simulink model "abssq04_fixpt8_32"  (R2021b)
settings: Solver=VariableStepAuto  StartTime=0.0  StopTime=99  RelTol=1e-3
undefined symbols (not defined in the file or in its folder): figd2104, xcu250
libraries: hdlBasic x720, vmcUtilities x1
(part 5 of 7)

== system abssq04_fixpt8_32/total32/Subsystem25bit ==
  rex : Inport
  imx : Inport  Port=2
  CMult1 : hdlBasic/CMult  const=cos(pi/4)  gui_display_data_type=Fixed-point  const_n_bits=25  const_bin_pt=24  float_type=Single  exp_bits=8  fraction_bits=24  en=off  latency=0  precision=Full  arith_type="Signed  (2's comp)"  n_bits=16  bin_pt=14  quantization=Truncate  overflow=Wrap  use_behavioral_HDL=off  mem_type=Distributed RAM  pipeline=off  XmcBlockStatus=1  maskContainerNames=tabcontainer1  block_type=cmult  block_config=sysgen:CMult_config
      settings: infoedit=[]
  CMult2 : hdlBasic/CMult  const=cos(pi/4)  gui_display_data_type=Fixed-point  const_n_bits=25  const_bin_pt=24  float_type=Single  exp_bits=8  fraction_bits=24  en=off  latency=0  precision=Full  arith_type="Signed  (2's comp)"  n_bits=16  bin_pt=14  quantization=Truncate  overflow=Wrap  use_behavioral_HDL=off  mem_type=Distributed RAM  pipeline=off  XmcBlockStatus=1  maskContainerNames=tabcontainer1  block_type=cmult  block_config=sysgen:CMult_config
      settings: infoedit=[]
  CMult3 : hdlBasic/CMult  const=1/sqrt(2)  gui_display_data_type=Fixed-point  const_n_bits=25  const_bin_pt=24  float_type=Single  exp_bits=8  fraction_bits=24  en=off  latency=0  precision=Full  arith_type="Signed  (2's comp)"  n_bits=16  bin_pt=14  quantization=Truncate  overflow=Wrap  use_behavioral_HDL=off  mem_type=Distributed RAM  pipeline=off  XmcBlockStatus=1  maskContainerNames=tabcontainer1  block_type=cmult  block_config=sysgen:CMult_config
      settings: infoedit=[]
  COS_PI : hdlBasic/Constant  Commented=on  const=cos(pi/4)  gui_display_data_type=Fixed-point  arith_type=Unsigned  n_bits=8  bin_pt=7  preci_type=Double  exp_width=8  frac_width=24  explicit_period=on  period=1  XmcBlockStatus=1  maskContainerNames=tabcontainer1  block_type=constant  block_config=sysgen:Constant_config
  Cast1 : hdlBasic/Convert  Commented=on  gui_display_data_type=Fixed-point  arith_type=Unsigned  n_bits=8  bin_pt=7  float_type=Double  exp_bits=8  fraction_bits=24  quantization="Round  (unbiased: +/- Inf)"  overflow=Saturate  en=off  latency=0  pipeline=on  XmcBlockStatus=1  maskContainerNames=group2  block_type=convert  block_config=sysgen:Convert_config
  Cast2 : hdlBasic/Convert  Commented=on  gui_display_data_type=Fixed-point  arith_type=Unsigned  n_bits=8  bin_pt=7  float_type=Double  exp_bits=8  fraction_bits=24  quantization="Round  (unbiased: +/- Inf)"  overflow=Saturate  en=off  latency=0  pipeline=on  XmcBlockStatus=1  maskContainerNames=group2  block_type=convert  block_config=sysgen:Convert_config
  Cast3 : hdlBasic/Convert  Commented=on  gui_display_data_type=Fixed-point  arith_type=Unsigned  n_bits=8  bin_pt=7  float_type=Double  exp_bits=8  fraction_bits=24  quantization="Round  (unbiased: +/- Inf)"  overflow=Saturate  en=off  latency=0  pipeline=on  XmcBlockStatus=1  maskContainerNames=group2  block_type=convert  block_config=sysgen:Convert_config
  Gate_In1 : hdlBasic/Gateway In  gui_display_data_type=Fixed-point  arith_type=Signed (2's comp)  n_bits=25  bin_pt=23  preci_type=Double  exp_width=8  frac_width=24  rows=1  columns=1  quantization=Truncate  overflow=Wrap  period=1  UseAsADC=off  ADCChannel='1'  interface=None  automatic_assignment=on  address_offset=hex2dec('00')  intf_name=''  intf_description=''  default_value=0  timing_constraint=None  locs_specified=off  LOCs={}  io_standard={}  inherit_from_input=off  hdl_port=on  XmcBlockStatus=1  maskContainerNames=group4  block_type=gatewayin  block_config=sysgen:gateway_in_config  block_width_w=590  block_height_w=620  block_width=640  block_height=850
  Gate_In2 : hdlBasic/Gateway In  gui_display_data_type=Fixed-point  arith_type=Signed (2's comp)  n_bits=25  bin_pt=23  preci_type=Double  exp_width=8  frac_width=24  rows=1  columns=1  quantization=Truncate  overflow=Wrap  period=1  UseAsADC=off  ADCChannel='1'  interface=None  automatic_assignment=on  address_offset=hex2dec('00')  intf_name=''  intf_description=''  default_value=0  timing_constraint=None  locs_specified=off  LOCs={}  io_standard={}  inherit_from_input=off  hdl_port=on  XmcBlockStatus=1  maskContainerNames=group4  block_type=gatewayin  block_config=sysgen:gateway_in_config  block_width_w=590  block_height_w=620  block_width=640  block_height=850
  Gate_out1 : hdlBasic/Gateway Out  inherit_from_input=off  hdl_port=on  rows=1  columns=1  UseAsDAC=off  DACChannel='1'  interface=None  automatic_assignment=on  address_offset=hex2dec('00')  intf_name=''  intf_description=''  timing_constraint=None  locs_specified=off  LOCs={}  io_standard={}  XmcBlockStatus=1  maskContainerNames=group4  block_type=gatewayout  block_config=sysgen:gateway_out_config  block_width_w=590  block_height_w=620  block_width=620  block_height=750
  Mux : hdlBasic/Mux  inputs=2  en=off  latency=0  precision=Full  arith_type=Unsigned  n_bits=16  bin_pt=14  quantization=Truncate  overflow=Wrap  XmcBlockStatus=1  maskContainerNames=tabcontainer1  block_type=mux  block_config=sysgen:Mux_config
  Scale1 : hdlBasic/Scale  scale_factor=-24  XmcBlockStatus=1  maskContainerNames=group1  block_type=scale  block_config=sysgen:Scale_config
  Scale2 : hdlBasic/Scale  scale_factor=-23  XmcBlockStatus=1  maskContainerNames=group1  block_type=scale  block_config=sysgen:Scale_config
  Scale3 : hdlBasic/Scale  scale_factor=-24  XmcBlockStatus=1  maskContainerNames=group1  block_type=scale  block_config=sysgen:Scale_config
  Slice1 : hdlBasic/Slice  nbits=8  boolean_output=off  mode=Two Bit Locations  bit1=-1  base1=MSB of Input  bit0=24  base0=LSB of Input  XmcBlockStatus=1  maskContainerNames=group1  block_type=slice  block_config=sysgen:Slice_config
  Slice2 : hdlBasic/Slice  nbits=24  boolean_output=off  mode=Upper Bit Location + Width  bit1=-3  base1=MSB of Input  bit0=7  base0=LSB of Input  XmcBlockStatus=1  maskContainerNames=group1  block_type=slice  block_config=sysgen:Slice_config
  Slice3 : hdlBasic/Slice  nbits=7  boolean_output=off  mode=Two Bit Locations  bit1=-5  base1=MSB of Input  bit0=23  base0=LSB of Input  XmcBlockStatus=1  maskContainerNames=group1  block_type=slice  block_config=sysgen:Slice_config
  abs{1..4} (4 alike) : hdlBasic/Absolute  precision=Full  arith_type=Unsigned  n_bits=16  bin_pt=14  quantization=Truncate  overflow=Wrap  en=off  latency=0  XmcBlockStatus=1  maskContainerNames=tabcontainer1  block_type=abs  block_config=sysgen:Abs_config
  addsub1 : hdlBasic/AddSub  mode=Subtraction  use_carryin=off  use_carryout=off  en=off  latency=0  precision=Full  arith_type="Signed  (2's comp)"  n_bits=35  bin_pt=32  quantization="Round  (unbiased: +/- Inf)"  overflow=Saturate  use_behavioral_HDL=off  hw_selection=Fabric  pipelined=on  XmcBlockStatus=1  maskContainerNames=tabcontainer1  block_type=addsub  block_config=sysgen:Addsub_config
  addsub2 : hdlBasic/AddSub  mode=Addition  use_carryin=off  use_carryout=off  en=off  latency=0  precision=Full  arith_type=Unsigned  n_bits=16  bin_pt=14  quantization="Round  (unbiased: +/- Inf)"  overflow=Saturate  use_behavioral_HDL=off  hw_selection=Fabric  pipelined=on  XmcBlockStatus=1  maskContainerNames=tabcontainer1  block_type=addsub  block_config=sysgen:Addsub_config
  addsub3 : hdlBasic/AddSub  mode=Addition  use_carryin=off  use_carryout=off  en=off  latency=0  precision=Full  arith_type=Unsigned  n_bits=16  bin_pt=14  quantization="Round  (unbiased: +/- Inf)"  overflow=Saturate  use_behavioral_HDL=off  hw_selection=Fabric  pipelined=on  XmcBlockStatus=1  maskContainerNames=tabcontainer1  block_type=addsub  block_config=sysgen:Addsub_config
  addsub4 : hdlBasic/AddSub  mode=Addition  use_carryin=off  use_carryout=off  en=off  latency=0  precision=Full  arith_type=Unsigned  n_bits=17  bin_pt=16  quantization="Round  (unbiased: +/- Inf)"  overflow=Saturate  use_behavioral_HDL=off  hw_selection=Fabric  pipelined=on  XmcBlockStatus=1  maskContainerNames=tabcontainer1  block_type=addsub  block_config=sysgen:Addsub_config
  bool1 : hdlBasic/Relational  mode=a<b  op_type=Bool  en=off  latency=0  XmcBlockStatus=1  maskContainerNames=tabcontainer1  block_type=relational  block_config=sysgen:Relational_config
  mult1 : hdlBasic/Mult  Commented=on  precision=Full  arith_type=Unsigned  n_bits=32  bin_pt=32  quantization="Round  (unbiased: +/- Inf)"  overflow=Saturate  en=off  latency=0  use_behavioral_HDL=off  opt=Area  use_embedded=off  optimum_pipeline=off  pipeline=on  use_rpm=on  placement_style=Triangular  XmcBlockStatus=1  maskContainerNames=group1  block_type=mult  block_config=sysgen:Mult_config
  mult2 : hdlBasic/Mult  Commented=on  precision=Full  arith_type=Unsigned  n_bits=32  bin_pt=32  quantization="Round  (unbiased: +/- Inf)"  overflow=Saturate  en=off  latency=0  use_behavioral_HDL=off  opt=Area  use_embedded=off  optimum_pipeline=off  pipeline=on  use_rpm=on  placement_style=Triangular  XmcBlockStatus=1  maskContainerNames=group1  block_type=mult  block_config=sysgen:Mult_config
  mult3 : hdlBasic/Mult  Commented=on  precision=Full  arith_type="Signed  (2's comp)"  n_bits=16  bin_pt=14  quantization="Round  (unbiased: +/- Inf)"  overflow=Saturate  en=off  latency=0  use_behavioral_HDL=off  opt=Area  use_embedded=off  optimum_pipeline=off  pipeline=on  use_rpm=on  placement_style=Triangular  XmcBlockStatus=1  maskContainerNames=group1  block_type=mult  block_config=sysgen:Mult_config
  Out1 : Outport
  wires:
  addsub1/1 -> abs1/1
  abs1/1 -> addsub3/1
  CMult1/1 -> addsub2/1, addsub1/1
  CMult2/1 -> addsub2/2, addsub1/2
  CMult3/1 -> Slice1/1
  Mux/1 -> CMult3/1
  imx/1 -> Gate_In2/1
  Gate_out1/1 -> Out1/1
  rex/1 -> Gate_In1/1
  Slice1/1 -> Scale1/1
  bool1/1 -> Mux/1
  addsub3/1 -> Slice3/1
  addsub4/1 -> Slice2/1
  addsub2/1 -> abs2/1
  Gate_In2/1 -> abs4/1, CMult2/1
  Gate_In1/1 -> CMult1/1, abs3/1
  abs2/1 -> addsub3/2
  abs3/1 -> addsub4/1
  abs4/1 -> addsub4/2
  Scale1/1 -> Gate_out1/1
  Slice2/1 -> Scale2/1
  Scale3/1 -> bool1/1, Mux/2
  Scale2/1 -> Mux/3, bool1/2
  Slice3/1 -> Scale3/1

== system abssq04_fixpt8_32/total32/Subsystem26bit ==
  rex : Inport
  imx : Inport  Port=2
  CMult1 : hdlBasic/CMult  const=cos(pi/4)  gui_display_data_type=Fixed-point  const_n_bits=26  const_bin_pt=25  float_type=Single  exp_bits=8  fraction_bits=24  en=off  latency=0  precision=Full  arith_type="Signed  (2's comp)"  n_bits=16  bin_pt=14  quantization=Truncate  overflow=Wrap  use_behavioral_HDL=off  mem_type=Distributed RAM  pipeline=off  XmcBlockStatus=1  maskContainerNames=tabcontainer1  block_type=cmult  block_config=sysgen:CMult_config
      settings: infoedit=[]
  CMult2 : hdlBasic/CMult  const=cos(pi/4)  gui_display_data_type=Fixed-point  const_n_bits=26  const_bin_pt=25  float_type=Single  exp_bits=8  fraction_bits=24  en=off  latency=0  precision=Full  arith_type="Signed  (2's comp)"  n_bits=16  bin_pt=14  quantization=Truncate  overflow=Wrap  use_behavioral_HDL=off  mem_type=Distributed RAM  pipeline=off  XmcBlockStatus=1  maskContainerNames=tabcontainer1  block_type=cmult  block_config=sysgen:CMult_config
      settings: infoedit=[]
  CMult3 : hdlBasic/CMult  const=1/sqrt(2)  gui_display_data_type=Fixed-point  const_n_bits=26  const_bin_pt=25  float_type=Single  exp_bits=8  fraction_bits=24  en=off  latency=0  precision=Full  arith_type="Signed  (2's comp)"  n_bits=16  bin_pt=14  quantization=Truncate  overflow=Wrap  use_behavioral_HDL=off  mem_type=Distributed RAM  pipeline=off  XmcBlockStatus=1  maskContainerNames=tabcontainer1  block_type=cmult  block_config=sysgen:CMult_config
      settings: infoedit=[]
  COS_PI : hdlBasic/Constant  Commented=on  const=cos(pi/4)  gui_display_data_type=Fixed-point  arith_type=Unsigned  n_bits=8  bin_pt=7  preci_type=Double  exp_width=8  frac_width=24  explicit_period=on  period=1  XmcBlockStatus=1  maskContainerNames=tabcontainer1  block_type=constant  block_config=sysgen:Constant_config
  Cast1 : hdlBasic/Convert  Commented=on  gui_display_data_type=Fixed-point  arith_type=Unsigned  n_bits=8  bin_pt=7  float_type=Double  exp_bits=8  fraction_bits=24  quantization="Round  (unbiased: +/- Inf)"  overflow=Saturate  en=off  latency=0  pipeline=on  XmcBlockStatus=1  maskContainerNames=group2  block_type=convert  block_config=sysgen:Convert_config
  Cast2 : hdlBasic/Convert  Commented=on  gui_display_data_type=Fixed-point  arith_type=Unsigned  n_bits=8  bin_pt=7  float_type=Double  exp_bits=8  fraction_bits=24  quantization="Round  (unbiased: +/- Inf)"  overflow=Saturate  en=off  latency=0  pipeline=on  XmcBlockStatus=1  maskContainerNames=group2  block_type=convert  block_config=sysgen:Convert_config
  Cast3 : hdlBasic/Convert  Commented=on  gui_display_data_type=Fixed-point  arith_type=Unsigned  n_bits=8  bin_pt=7  float_type=Double  exp_bits=8  fraction_bits=24  quantization="Round  (unbiased: +/- Inf)"  overflow=Saturate  en=off  latency=0  pipeline=on  XmcBlockStatus=1  maskContainerNames=group2  block_type=convert  block_config=sysgen:Convert_config
  Gate_In1 : hdlBasic/Gateway In  gui_display_data_type=Fixed-point  arith_type=Signed (2's comp)  n_bits=26  bin_pt=24  preci_type=Double  exp_width=8  frac_width=24  rows=1  columns=1  quantization=Truncate  overflow=Wrap  period=1  UseAsADC=off  ADCChannel='1'  interface=None  automatic_assignment=on  address_offset=hex2dec('00')  intf_name=''  intf_description=''  default_value=0  timing_constraint=None  locs_specified=off  LOCs={}  io_standard={}  inherit_from_input=off  hdl_port=on  XmcBlockStatus=1  maskContainerNames=group4  block_type=gatewayin  block_config=sysgen:gateway_in_config  block_width_w=590  block_height_w=620  block_width=640  block_height=850
  Gate_In2 : hdlBasic/Gateway In  gui_display_data_type=Fixed-point  arith_type=Signed (2's comp)  n_bits=26  bin_pt=24  preci_type=Double  exp_width=8  frac_width=24  rows=1  columns=1  quantization=Truncate  overflow=Wrap  period=1  UseAsADC=off  ADCChannel='1'  interface=None  automatic_assignment=on  address_offset=hex2dec('00')  intf_name=''  intf_description=''  default_value=0  timing_constraint=None  locs_specified=off  LOCs={}  io_standard={}  inherit_from_input=off  hdl_port=on  XmcBlockStatus=1  maskContainerNames=group4  block_type=gatewayin  block_config=sysgen:gateway_in_config  block_width_w=590  block_height_w=620  block_width=640  block_height=850
  Gate_out1 : hdlBasic/Gateway Out  inherit_from_input=off  hdl_port=on  rows=1  columns=1  UseAsDAC=off  DACChannel='1'  interface=None  automatic_assignment=on  address_offset=hex2dec('00')  intf_name=''  intf_description=''  timing_constraint=None  locs_specified=off  LOCs={}  io_standard={}  XmcBlockStatus=1  maskContainerNames=group4  block_type=gatewayout  block_config=sysgen:gateway_out_config  block_width_w=590  block_height_w=620  block_width=620  block_height=750
  Mux : hdlBasic/Mux  inputs=2  en=off  latency=0  precision=Full  arith_type=Unsigned  n_bits=16  bin_pt=14  quantization=Truncate  overflow=Wrap  XmcBlockStatus=1  maskContainerNames=tabcontainer1  block_type=mux  block_config=sysgen:Mux_config
  Scale1 : hdlBasic/Scale  scale_factor=-25  XmcBlockStatus=1  maskContainerNames=group1  block_type=scale  block_config=sysgen:Scale_config
  Scale2 : hdlBasic/Scale  scale_factor=-24  XmcBlockStatus=1  maskContainerNames=group1  block_type=scale  block_config=sysgen:Scale_config
  Scale3 : hdlBasic/Scale  scale_factor=-25  XmcBlockStatus=1  maskContainerNames=group1  block_type=scale  block_config=sysgen:Scale_config
  Slice1 : hdlBasic/Slice  nbits=8  boolean_output=off  mode=Two Bit Locations  bit1=-1  base1=MSB of Input  bit0=25  base0=LSB of Input  XmcBlockStatus=1  maskContainerNames=group1  block_type=slice  block_config=sysgen:Slice_config
  Slice2 : hdlBasic/Slice  nbits=25  boolean_output=off  mode=Upper Bit Location + Width  bit1=-3  base1=MSB of Input  bit0=7  base0=LSB of Input  XmcBlockStatus=1  maskContainerNames=group1  block_type=slice  block_config=sysgen:Slice_config
  Slice3 : hdlBasic/Slice  nbits=7  boolean_output=off  mode=Two Bit Locations  bit1=-5  base1=MSB of Input  bit0=24  base0=LSB of Input  XmcBlockStatus=1  maskContainerNames=group1  block_type=slice  block_config=sysgen:Slice_config
  abs{1..4} (4 alike) : hdlBasic/Absolute  precision=Full  arith_type=Unsigned  n_bits=16  bin_pt=14  quantization=Truncate  overflow=Wrap  en=off  latency=0  XmcBlockStatus=1  maskContainerNames=tabcontainer1  block_type=abs  block_config=sysgen:Abs_config
  addsub1 : hdlBasic/AddSub  mode=Subtraction  use_carryin=off  use_carryout=off  en=off  latency=0  precision=Full  arith_type="Signed  (2's comp)"  n_bits=35  bin_pt=32  quantization="Round  (unbiased: +/- Inf)"  overflow=Saturate  use_behavioral_HDL=off  hw_selection=Fabric  pipelined=on  XmcBlockStatus=1  maskContainerNames=tabcontainer1  block_type=addsub  block_config=sysgen:Addsub_config
  addsub2 : hdlBasic/AddSub  mode=Addition  use_carryin=off  use_carryout=off  en=off  latency=0  precision=Full  arith_type=Unsigned  n_bits=16  bin_pt=14  quantization="Round  (unbiased: +/- Inf)"  overflow=Saturate  use_behavioral_HDL=off  hw_selection=Fabric  pipelined=on  XmcBlockStatus=1  maskContainerNames=tabcontainer1  block_type=addsub  block_config=sysgen:Addsub_config
  addsub3 : hdlBasic/AddSub  mode=Addition  use_carryin=off  use_carryout=off  en=off  latency=0  precision=Full  arith_type=Unsigned  n_bits=16  bin_pt=14  quantization="Round  (unbiased: +/- Inf)"  overflow=Saturate  use_behavioral_HDL=off  hw_selection=Fabric  pipelined=on  XmcBlockStatus=1  maskContainerNames=tabcontainer1  block_type=addsub  block_config=sysgen:Addsub_config
  addsub4 : hdlBasic/AddSub  mode=Addition  use_carryin=off  use_carryout=off  en=off  latency=0  precision=Full  arith_type=Unsigned  n_bits=17  bin_pt=16  quantization="Round  (unbiased: +/- Inf)"  overflow=Saturate  use_behavioral_HDL=off  hw_selection=Fabric  pipelined=on  XmcBlockStatus=1  maskContainerNames=tabcontainer1  block_type=addsub  block_config=sysgen:Addsub_config
  bool1 : hdlBasic/Relational  mode=a<b  op_type=Bool  en=off  latency=0  XmcBlockStatus=1  maskContainerNames=tabcontainer1  block_type=relational  block_config=sysgen:Relational_config
  mult1 : hdlBasic/Mult  Commented=on  precision=Full  arith_type=Unsigned  n_bits=32  bin_pt=32  quantization="Round  (unbiased: +/- Inf)"  overflow=Saturate  en=off  latency=0  use_behavioral_HDL=off  opt=Area  use_embedded=off  optimum_pipeline=off  pipeline=on  use_rpm=on  placement_style=Triangular  XmcBlockStatus=1  maskContainerNames=group1  block_type=mult  block_config=sysgen:Mult_config
  mult2 : hdlBasic/Mult  Commented=on  precision=Full  arith_type=Unsigned  n_bits=32  bin_pt=32  quantization="Round  (unbiased: +/- Inf)"  overflow=Saturate  en=off  latency=0  use_behavioral_HDL=off  opt=Area  use_embedded=off  optimum_pipeline=off  pipeline=on  use_rpm=on  placement_style=Triangular  XmcBlockStatus=1  maskContainerNames=group1  block_type=mult  block_config=sysgen:Mult_config
  mult3 : hdlBasic/Mult  Commented=on  precision=Full  arith_type="Signed  (2's comp)"  n_bits=16  bin_pt=14  quantization="Round  (unbiased: +/- Inf)"  overflow=Saturate  en=off  latency=0  use_behavioral_HDL=off  opt=Area  use_embedded=off  optimum_pipeline=off  pipeline=on  use_rpm=on  placement_style=Triangular  XmcBlockStatus=1  maskContainerNames=group1  block_type=mult  block_config=sysgen:Mult_config
  Out1 : Outport
  wires:
  addsub1/1 -> abs1/1
  abs1/1 -> addsub3/1
  CMult1/1 -> addsub2/1, addsub1/1
  CMult2/1 -> addsub2/2, addsub1/2
  CMult3/1 -> Slice1/1
  Mux/1 -> CMult3/1
  imx/1 -> Gate_In2/1
  Gate_out1/1 -> Out1/1
  rex/1 -> Gate_In1/1
  Slice1/1 -> Scale1/1
  bool1/1 -> Mux/1
  addsub3/1 -> Slice3/1
  addsub4/1 -> Slice2/1
  addsub2/1 -> abs2/1
  Gate_In2/1 -> abs4/1, CMult2/1
  Gate_In1/1 -> CMult1/1, abs3/1
  abs2/1 -> addsub3/2
  abs3/1 -> addsub4/1
  abs4/1 -> addsub4/2
  Scale1/1 -> Gate_out1/1
  Slice2/1 -> Scale2/1
  Scale3/1 -> bool1/1, Mux/2
  Scale2/1 -> Mux/3, bool1/2
  Slice3/1 -> Scale3/1

== system abssq04_fixpt8_32/total32/Subsystem27bit ==
  rex : Inport
  imx : Inport  Port=2
  CMult1 : hdlBasic/CMult  const=cos(pi/4)  gui_display_data_type=Fixed-point  const_n_bits=27  const_bin_pt=26  float_type=Single  exp_bits=8  fraction_bits=24  en=off  latency=0  precision=Full  arith_type="Signed  (2's comp)"  n_bits=16  bin_pt=14  quantization=Truncate  overflow=Wrap  use_behavioral_HDL=off  mem_type=Distributed RAM  pipeline=off  XmcBlockStatus=1  maskContainerNames=tabcontainer1  block_type=cmult  block_config=sysgen:CMult_config
      settings: infoedit=[]
  CMult2 : hdlBasic/CMult  const=cos(pi/4)  gui_display_data_type=Fixed-point  const_n_bits=27  const_bin_pt=26  float_type=Single  exp_bits=8  fraction_bits=24  en=off  latency=0  precision=Full  arith_type="Signed  (2's comp)"  n_bits=16  bin_pt=14  quantization=Truncate  overflow=Wrap  use_behavioral_HDL=off  mem_type=Distributed RAM  pipeline=off  XmcBlockStatus=1  maskContainerNames=tabcontainer1  block_type=cmult  block_config=sysgen:CMult_config
      settings: infoedit=[]
  CMult3 : hdlBasic/CMult  const=1/sqrt(2)  gui_display_data_type=Fixed-point  const_n_bits=27  const_bin_pt=26  float_type=Single  exp_bits=8  fraction_bits=24  en=off  latency=0  precision=Full  arith_type="Signed  (2's comp)"  n_bits=16  bin_pt=14  quantization=Truncate  overflow=Wrap  use_behavioral_HDL=off  mem_type=Distributed RAM  pipeline=off  XmcBlockStatus=1  maskContainerNames=tabcontainer1  block_type=cmult  block_config=sysgen:CMult_config
      settings: infoedit=[]
  COS_PI : hdlBasic/Constant  Commented=on  const=cos(pi/4)  gui_display_data_type=Fixed-point  arith_type=Unsigned  n_bits=8  bin_pt=7  preci_type=Double  exp_width=8  frac_width=24  explicit_period=on  period=1  XmcBlockStatus=1  maskContainerNames=tabcontainer1  block_type=constant  block_config=sysgen:Constant_config
  Cast1 : hdlBasic/Convert  Commented=on  gui_display_data_type=Fixed-point  arith_type=Unsigned  n_bits=8  bin_pt=7  float_type=Double  exp_bits=8  fraction_bits=24  quantization="Round  (unbiased: +/- Inf)"  overflow=Saturate  en=off  latency=0  pipeline=on  XmcBlockStatus=1  maskContainerNames=group2  block_type=convert  block_config=sysgen:Convert_config
  Cast2 : hdlBasic/Convert  Commented=on  gui_display_data_type=Fixed-point  arith_type=Unsigned  n_bits=8  bin_pt=7  float_type=Double  exp_bits=8  fraction_bits=24  quantization="Round  (unbiased: +/- Inf)"  overflow=Saturate  en=off  latency=0  pipeline=on  XmcBlockStatus=1  maskContainerNames=group2  block_type=convert  block_config=sysgen:Convert_config
  Cast3 : hdlBasic/Convert  Commented=on  gui_display_data_type=Fixed-point  arith_type=Unsigned  n_bits=8  bin_pt=7  float_type=Double  exp_bits=8  fraction_bits=24  quantization="Round  (unbiased: +/- Inf)"  overflow=Saturate  en=off  latency=0  pipeline=on  XmcBlockStatus=1  maskContainerNames=group2  block_type=convert  block_config=sysgen:Convert_config
  Gate_In1 : hdlBasic/Gateway In  gui_display_data_type=Fixed-point  arith_type=Signed (2's comp)  n_bits=27  bin_pt=25  preci_type=Double  exp_width=8  frac_width=24  rows=1  columns=1  quantization=Truncate  overflow=Wrap  period=1  UseAsADC=off  ADCChannel='1'  interface=None  automatic_assignment=on  address_offset=hex2dec('00')  intf_name=''  intf_description=''  default_value=0  timing_constraint=None  locs_specified=off  LOCs={}  io_standard={}  inherit_from_input=off  hdl_port=on  XmcBlockStatus=1  maskContainerNames=group4  block_type=gatewayin  block_config=sysgen:gateway_in_config  block_width_w=590  block_height_w=620  block_width=640  block_height=850
  Gate_In2 : hdlBasic/Gateway In  gui_display_data_type=Fixed-point  arith_type=Signed (2's comp)  n_bits=27  bin_pt=25  preci_type=Double  exp_width=8  frac_width=24  rows=1  columns=1  quantization=Truncate  overflow=Wrap  period=1  UseAsADC=off  ADCChannel='1'  interface=None  automatic_assignment=on  address_offset=hex2dec('00')  intf_name=''  intf_description=''  default_value=0  timing_constraint=None  locs_specified=off  LOCs={}  io_standard={}  inherit_from_input=off  hdl_port=on  XmcBlockStatus=1  maskContainerNames=group4  block_type=gatewayin  block_config=sysgen:gateway_in_config  block_width_w=590  block_height_w=620  block_width=640  block_height=850
  Gate_out1 : hdlBasic/Gateway Out  inherit_from_input=off  hdl_port=on  rows=1  columns=1  UseAsDAC=off  DACChannel='1'  interface=None  automatic_assignment=on  address_offset=hex2dec('00')  intf_name=''  intf_description=''  timing_constraint=None  locs_specified=off  LOCs={}  io_standard={}  XmcBlockStatus=1  maskContainerNames=group4  block_type=gatewayout  block_config=sysgen:gateway_out_config  block_width_w=590  block_height_w=620  block_width=620  block_height=750
  Mux : hdlBasic/Mux  inputs=2  en=off  latency=0  precision=Full  arith_type=Unsigned  n_bits=16  bin_pt=14  quantization=Truncate  overflow=Wrap  XmcBlockStatus=1  maskContainerNames=tabcontainer1  block_type=mux  block_config=sysgen:Mux_config
  Scale1 : hdlBasic/Scale  scale_factor=-26  XmcBlockStatus=1  maskContainerNames=group1  block_type=scale  block_config=sysgen:Scale_config
  Scale2 : hdlBasic/Scale  scale_factor=-25  XmcBlockStatus=1  maskContainerNames=group1  block_type=scale  block_config=sysgen:Scale_config
  Scale3 : hdlBasic/Scale  scale_factor=-26  XmcBlockStatus=1  maskContainerNames=group1  block_type=scale  block_config=sysgen:Scale_config
  Slice1 : hdlBasic/Slice  nbits=8  boolean_output=off  mode=Two Bit Locations  bit1=-1  base1=MSB of Input  bit0=26  base0=LSB of Input  XmcBlockStatus=1  maskContainerNames=group1  block_type=slice  block_config=sysgen:Slice_config
  Slice2 : hdlBasic/Slice  nbits=26  boolean_output=off  mode=Upper Bit Location + Width  bit1=-3  base1=MSB of Input  bit0=7  base0=LSB of Input  XmcBlockStatus=1  maskContainerNames=group1  block_type=slice  block_config=sysgen:Slice_config
  Slice3 : hdlBasic/Slice  nbits=7  boolean_output=off  mode=Two Bit Locations  bit1=-5  base1=MSB of Input  bit0=25  base0=LSB of Input  XmcBlockStatus=1  maskContainerNames=group1  block_type=slice  block_config=sysgen:Slice_config
  abs{1..4} (4 alike) : hdlBasic/Absolute  precision=Full  arith_type=Unsigned  n_bits=16  bin_pt=14  quantization=Truncate  overflow=Wrap  en=off  latency=0  XmcBlockStatus=1  maskContainerNames=tabcontainer1  block_type=abs  block_config=sysgen:Abs_config
  addsub1 : hdlBasic/AddSub  mode=Subtraction  use_carryin=off  use_carryout=off  en=off  latency=0  precision=Full  arith_type="Signed  (2's comp)"  n_bits=35  bin_pt=32  quantization="Round  (unbiased: +/- Inf)"  overflow=Saturate  use_behavioral_HDL=off  hw_selection=Fabric  pipelined=on  XmcBlockStatus=1  maskContainerNames=tabcontainer1  block_type=addsub  block_config=sysgen:Addsub_config
  addsub2 : hdlBasic/AddSub  mode=Addition  use_carryin=off  use_carryout=off  en=off  latency=0  precision=Full  arith_type=Unsigned  n_bits=16  bin_pt=14  quantization="Round  (unbiased: +/- Inf)"  overflow=Saturate  use_behavioral_HDL=off  hw_selection=Fabric  pipelined=on  XmcBlockStatus=1  maskContainerNames=tabcontainer1  block_type=addsub  block_config=sysgen:Addsub_config
  addsub3 : hdlBasic/AddSub  mode=Addition  use_carryin=off  use_carryout=off  en=off  latency=0  precision=Full  arith_type=Unsigned  n_bits=16  bin_pt=14  quantization="Round  (unbiased: +/- Inf)"  overflow=Saturate  use_behavioral_HDL=off  hw_selection=Fabric  pipelined=on  XmcBlockStatus=1  maskContainerNames=tabcontainer1  block_type=addsub  block_config=sysgen:Addsub_config
  addsub4 : hdlBasic/AddSub  mode=Addition  use_carryin=off  use_carryout=off  en=off  latency=0  precision=Full  arith_type=Unsigned  n_bits=17  bin_pt=16  quantization="Round  (unbiased: +/- Inf)"  overflow=Saturate  use_behavioral_HDL=off  hw_selection=Fabric  pipelined=on  XmcBlockStatus=1  maskContainerNames=tabcontainer1  block_type=addsub  block_config=sysgen:Addsub_config
  bool1 : hdlBasic/Relational  mode=a<b  op_type=Bool  en=off  latency=0  XmcBlockStatus=1  maskContainerNames=tabcontainer1  block_type=relational  block_config=sysgen:Relational_config
  mult1 : hdlBasic/Mult  Commented=on  precision=Full  arith_type=Unsigned  n_bits=32  bin_pt=32  quantization="Round  (unbiased: +/- Inf)"  overflow=Saturate  en=off  latency=0  use_behavioral_HDL=off  opt=Area  use_embedded=off  optimum_pipeline=off  pipeline=on  use_rpm=on  placement_style=Triangular  XmcBlockStatus=1  maskContainerNames=group1  block_type=mult  block_config=sysgen:Mult_config
  mult2 : hdlBasic/Mult  Commented=on  precision=Full  arith_type=Unsigned  n_bits=32  bin_pt=32  quantization="Round  (unbiased: +/- Inf)"  overflow=Saturate  en=off  latency=0  use_behavioral_HDL=off  opt=Area  use_embedded=off  optimum_pipeline=off  pipeline=on  use_rpm=on  placement_style=Triangular  XmcBlockStatus=1  maskContainerNames=group1  block_type=mult  block_config=sysgen:Mult_config
  mult3 : hdlBasic/Mult  Commented=on  precision=Full  arith_type="Signed  (2's comp)"  n_bits=16  bin_pt=14  quantization="Round  (unbiased: +/- Inf)"  overflow=Saturate  en=off  latency=0  use_behavioral_HDL=off  opt=Area  use_embedded=off  optimum_pipeline=off  pipeline=on  use_rpm=on  placement_style=Triangular  XmcBlockStatus=1  maskContainerNames=group1  block_type=mult  block_config=sysgen:Mult_config
  Out1 : Outport
  wires:
  addsub1/1 -> abs1/1
  abs1/1 -> addsub3/1
  CMult1/1 -> addsub2/1, addsub1/1
  CMult2/1 -> addsub2/2, addsub1/2
  CMult3/1 -> Slice1/1
  Mux/1 -> CMult3/1
  imx/1 -> Gate_In2/1
  Gate_out1/1 -> Out1/1
  rex/1 -> Gate_In1/1
  Slice1/1 -> Scale1/1
  bool1/1 -> Mux/1
  addsub3/1 -> Slice3/1
  addsub4/1 -> Slice2/1
  addsub2/1 -> abs2/1
  Gate_In2/1 -> abs4/1, CMult2/1
  Gate_In1/1 -> CMult1/1, abs3/1
  abs2/1 -> addsub3/2
  abs3/1 -> addsub4/1
  abs4/1 -> addsub4/2
  Scale1/1 -> Gate_out1/1
  Slice2/1 -> Scale2/1
  Scale3/1 -> bool1/1, Mux/2
  Scale2/1 -> Mux/3, bool1/2
  Slice3/1 -> Scale3/1

== system abssq04_fixpt8_32/total32/Subsystem28bit ==
  rex : Inport
  imx : Inport  Port=2
  CMult1 : hdlBasic/CMult  const=cos(pi/4)  gui_display_data_type=Fixed-point  const_n_bits=28  const_bin_pt=27  float_type=Single  exp_bits=8  fraction_bits=24  en=off  latency=0  precision=Full  arith_type="Signed  (2's comp)"  n_bits=16  bin_pt=14  quantization=Truncate  overflow=Wrap  use_behavioral_HDL=off  mem_type=Distributed RAM  pipeline=off  XmcBlockStatus=1  maskContainerNames=tabcontainer1  block_type=cmult  block_config=sysgen:CMult_config
      settings: infoedit=[]
  CMult2 : hdlBasic/CMult  const=cos(pi/4)  gui_display_data_type=Fixed-point  const_n_bits=28  const_bin_pt=27  float_type=Single  exp_bits=8  fraction_bits=24  en=off  latency=0  precision=Full  arith_type="Signed  (2's comp)"  n_bits=16  bin_pt=14  quantization=Truncate  overflow=Wrap  use_behavioral_HDL=off  mem_type=Distributed RAM  pipeline=off  XmcBlockStatus=1  maskContainerNames=tabcontainer1  block_type=cmult  block_config=sysgen:CMult_config
      settings: infoedit=[]
  CMult3 : hdlBasic/CMult  const=1/sqrt(2)  gui_display_data_type=Fixed-point  const_n_bits=28  const_bin_pt=27  float_type=Single  exp_bits=8  fraction_bits=24  en=off  latency=0  precision=Full  arith_type="Signed  (2's comp)"  n_bits=16  bin_pt=14  quantization=Truncate  overflow=Wrap  use_behavioral_HDL=off  mem_type=Distributed RAM  pipeline=off  XmcBlockStatus=1  maskContainerNames=tabcontainer1  block_type=cmult  block_config=sysgen:CMult_config
      settings: infoedit=[]
  COS_PI : hdlBasic/Constant  Commented=on  const=cos(pi/4)  gui_display_data_type=Fixed-point  arith_type=Unsigned  n_bits=8  bin_pt=7  preci_type=Double  exp_width=8  frac_width=24  explicit_period=on  period=1  XmcBlockStatus=1  maskContainerNames=tabcontainer1  block_type=constant  block_config=sysgen:Constant_config
  Cast1 : hdlBasic/Convert  Commented=on  gui_display_data_type=Fixed-point  arith_type=Unsigned  n_bits=8  bin_pt=7  float_type=Double  exp_bits=8  fraction_bits=24  quantization="Round  (unbiased: +/- Inf)"  overflow=Saturate  en=off  latency=0  pipeline=on  XmcBlockStatus=1  maskContainerNames=group2  block_type=convert  block_config=sysgen:Convert_config
  Cast2 : hdlBasic/Convert  Commented=on  gui_display_data_type=Fixed-point  arith_type=Unsigned  n_bits=8  bin_pt=7  float_type=Double  exp_bits=8  fraction_bits=24  quantization="Round  (unbiased: +/- Inf)"  overflow=Saturate  en=off  latency=0  pipeline=on  XmcBlockStatus=1  maskContainerNames=group2  block_type=convert  block_config=sysgen:Convert_config
  Cast3 : hdlBasic/Convert  Commented=on  gui_display_data_type=Fixed-point  arith_type=Unsigned  n_bits=8  bin_pt=7  float_type=Double  exp_bits=8  fraction_bits=24  quantization="Round  (unbiased: +/- Inf)"  overflow=Saturate  en=off  latency=0  pipeline=on  XmcBlockStatus=1  maskContainerNames=group2  block_type=convert  block_config=sysgen:Convert_config
  Gate_In1 : hdlBasic/Gateway In  gui_display_data_type=Fixed-point  arith_type=Signed (2's comp)  n_bits=28  bin_pt=26  preci_type=Double  exp_width=8  frac_width=24  rows=1  columns=1  quantization=Truncate  overflow=Wrap  period=1  UseAsADC=off  ADCChannel='1'  interface=None  automatic_assignment=on  address_offset=hex2dec('00')  intf_name=''  intf_description=''  default_value=0  timing_constraint=None  locs_specified=off  LOCs={}  io_standard={}  inherit_from_input=off  hdl_port=on  XmcBlockStatus=1  maskContainerNames=group4  block_type=gatewayin  block_config=sysgen:gateway_in_config  block_width_w=590  block_height_w=620  block_width=640  block_height=850
  Gate_In2 : hdlBasic/Gateway In  gui_display_data_type=Fixed-point  arith_type=Signed (2's comp)  n_bits=28  bin_pt=26  preci_type=Double  exp_width=8  frac_width=24  rows=1  columns=1  quantization=Truncate  overflow=Wrap  period=1  UseAsADC=off  ADCChannel='1'  interface=None  automatic_assignment=on  address_offset=hex2dec('00')  intf_name=''  intf_description=''  default_value=0  timing_constraint=None  locs_specified=off  LOCs={}  io_standard={}  inherit_from_input=off  hdl_port=on  XmcBlockStatus=1  maskContainerNames=group4  block_type=gatewayin  block_config=sysgen:gateway_in_config  block_width_w=590  block_height_w=620  block_width=640  block_height=850
  Gate_out1 : hdlBasic/Gateway Out  inherit_from_input=off  hdl_port=on  rows=1  columns=1  UseAsDAC=off  DACChannel='1'  interface=None  automatic_assignment=on  address_offset=hex2dec('00')  intf_name=''  intf_description=''  timing_constraint=None  locs_specified=off  LOCs={}  io_standard={}  XmcBlockStatus=1  maskContainerNames=group4  block_type=gatewayout  block_config=sysgen:gateway_out_config  block_width_w=590  block_height_w=620  block_width=620  block_height=750
  Mux : hdlBasic/Mux  inputs=2  en=off  latency=0  precision=Full  arith_type=Unsigned  n_bits=16  bin_pt=14  quantization=Truncate  overflow=Wrap  XmcBlockStatus=1  maskContainerNames=tabcontainer1  block_type=mux  block_config=sysgen:Mux_config
  Scale1 : hdlBasic/Scale  scale_factor=-27  XmcBlockStatus=1  maskContainerNames=group1  block_type=scale  block_config=sysgen:Scale_config
  Scale2 : hdlBasic/Scale  scale_factor=-26  XmcBlockStatus=1  maskContainerNames=group1  block_type=scale  block_config=sysgen:Scale_config
  Scale3 : hdlBasic/Scale  scale_factor=-27  XmcBlockStatus=1  maskContainerNames=group1  block_type=scale  block_config=sysgen:Scale_config
  Slice1 : hdlBasic/Slice  nbits=8  boolean_output=off  mode=Two Bit Locations  bit1=-1  base1=MSB of Input  bit0=27  base0=LSB of Input  XmcBlockStatus=1  maskContainerNames=group1  block_type=slice  block_config=sysgen:Slice_config
  Slice2 : hdlBasic/Slice  nbits=27  boolean_output=off  mode=Upper Bit Location + Width  bit1=-3  base1=MSB of Input  bit0=7  base0=LSB of Input  XmcBlockStatus=1  maskContainerNames=group1  block_type=slice  block_config=sysgen:Slice_config
  Slice3 : hdlBasic/Slice  nbits=7  boolean_output=off  mode=Two Bit Locations  bit1=-5  base1=MSB of Input  bit0=26  base0=LSB of Input  XmcBlockStatus=1  maskContainerNames=group1  block_type=slice  block_config=sysgen:Slice_config
  abs{1..4} (4 alike) : hdlBasic/Absolute  precision=Full  arith_type=Unsigned  n_bits=16  bin_pt=14  quantization=Truncate  overflow=Wrap  en=off  latency=0  XmcBlockStatus=1  maskContainerNames=tabcontainer1  block_type=abs  block_config=sysgen:Abs_config
  addsub1 : hdlBasic/AddSub  mode=Subtraction  use_carryin=off  use_carryout=off  en=off  latency=0  precision=Full  arith_type="Signed  (2's comp)"  n_bits=35  bin_pt=32  quantization="Round  (unbiased: +/- Inf)"  overflow=Saturate  use_behavioral_HDL=off  hw_selection=Fabric  pipelined=on  XmcBlockStatus=1  maskContainerNames=tabcontainer1  block_type=addsub  block_config=sysgen:Addsub_config
  addsub2 : hdlBasic/AddSub  mode=Addition  use_carryin=off  use_carryout=off  en=off  latency=0  precision=Full  arith_type=Unsigned  n_bits=16  bin_pt=14  quantization="Round  (unbiased: +/- Inf)"  overflow=Saturate  use_behavioral_HDL=off  hw_selection=Fabric  pipelined=on  XmcBlockStatus=1  maskContainerNames=tabcontainer1  block_type=addsub  block_config=sysgen:Addsub_config
  addsub3 : hdlBasic/AddSub  mode=Addition  use_carryin=off  use_carryout=off  en=off  latency=0  precision=Full  arith_type=Unsigned  n_bits=16  bin_pt=14  quantization="Round  (unbiased: +/- Inf)"  overflow=Saturate  use_behavioral_HDL=off  hw_selection=Fabric  pipelined=on  XmcBlockStatus=1  maskContainerNames=tabcontainer1  block_type=addsub  block_config=sysgen:Addsub_config
  addsub4 : hdlBasic/AddSub  mode=Addition  use_carryin=off  use_carryout=off  en=off  latency=0  precision=Full  arith_type=Unsigned  n_bits=17  bin_pt=16  quantization="Round  (unbiased: +/- Inf)"  overflow=Saturate  use_behavioral_HDL=off  hw_selection=Fabric  pipelined=on  XmcBlockStatus=1  maskContainerNames=tabcontainer1  block_type=addsub  block_config=sysgen:Addsub_config
  bool1 : hdlBasic/Relational  mode=a<b  op_type=Bool  en=off  latency=0  XmcBlockStatus=1  maskContainerNames=tabcontainer1  block_type=relational  block_config=sysgen:Relational_config
  mult1 : hdlBasic/Mult  Commented=on  precision=Full  arith_type=Unsigned  n_bits=32  bin_pt=32  quantization="Round  (unbiased: +/- Inf)"  overflow=Saturate  en=off  latency=0  use_behavioral_HDL=off  opt=Area  use_embedded=off  optimum_pipeline=off  pipeline=on  use_rpm=on  placement_style=Triangular  XmcBlockStatus=1  maskContainerNames=group1  block_type=mult  block_config=sysgen:Mult_config
  mult2 : hdlBasic/Mult  Commented=on  precision=Full  arith_type=Unsigned  n_bits=32  bin_pt=32  quantization="Round  (unbiased: +/- Inf)"  overflow=Saturate  en=off  latency=0  use_behavioral_HDL=off  opt=Area  use_embedded=off  optimum_pipeline=off  pipeline=on  use_rpm=on  placement_style=Triangular  XmcBlockStatus=1  maskContainerNames=group1  block_type=mult  block_config=sysgen:Mult_config
  mult3 : hdlBasic/Mult  Commented=on  precision=Full  arith_type="Signed  (2's comp)"  n_bits=16  bin_pt=14  quantization="Round  (unbiased: +/- Inf)"  overflow=Saturate  en=off  latency=0  use_behavioral_HDL=off  opt=Area  use_embedded=off  optimum_pipeline=off  pipeline=on  use_rpm=on  placement_style=Triangular  XmcBlockStatus=1  maskContainerNames=group1  block_type=mult  block_config=sysgen:Mult_config
  Out1 : Outport
  wires:
  addsub1/1 -> abs1/1
  abs1/1 -> addsub3/1
  CMult1/1 -> addsub2/1, addsub1/1
  CMult2/1 -> addsub2/2, addsub1/2
  CMult3/1 -> Slice1/1
  Mux/1 -> CMult3/1
  imx/1 -> Gate_In2/1
  Gate_out1/1 -> Out1/1
  rex/1 -> Gate_In1/1
  Slice1/1 -> Scale1/1
  bool1/1 -> Mux/1
  addsub3/1 -> Slice3/1
  addsub4/1 -> Slice2/1
  addsub2/1 -> abs2/1
  Gate_In2/1 -> abs4/1, CMult2/1
  Gate_In1/1 -> CMult1/1, abs3/1
  abs2/1 -> addsub3/2
  abs3/1 -> addsub4/1
  abs4/1 -> addsub4/2
  Scale1/1 -> Gate_out1/1
  Slice2/1 -> Scale2/1
  Scale3/1 -> bool1/1, Mux/2
  Scale2/1 -> Mux/3, bool1/2
  Slice3/1 -> Scale3/1

== system abssq04_fixpt8_32/total32/Subsystem29bit ==
  rex : Inport
  imx : Inport  Port=2
  CMult1 : hdlBasic/CMult  const=cos(pi/4)  gui_display_data_type=Fixed-point  const_n_bits=29  const_bin_pt=28  float_type=Single  exp_bits=8  fraction_bits=24  en=off  latency=0  precision=Full  arith_type="Signed  (2's comp)"  n_bits=16  bin_pt=14  quantization=Truncate  overflow=Wrap  use_behavioral_HDL=off  mem_type=Distributed RAM  pipeline=off  XmcBlockStatus=1  maskContainerNames=tabcontainer1  block_type=cmult  block_config=sysgen:CMult_config
      settings: infoedit=[]
  CMult2 : hdlBasic/CMult  const=cos(pi/4)  gui_display_data_type=Fixed-point  const_n_bits=29  const_bin_pt=28  float_type=Single  exp_bits=8  fraction_bits=24  en=off  latency=0  precision=Full  arith_type="Signed  (2's comp)"  n_bits=16  bin_pt=14  quantization=Truncate  overflow=Wrap  use_behavioral_HDL=off  mem_type=Distributed RAM  pipeline=off  XmcBlockStatus=1  maskContainerNames=tabcontainer1  block_type=cmult  block_config=sysgen:CMult_config
      settings: infoedit=[]
  CMult3 : hdlBasic/CMult  const=1/sqrt(2)  gui_display_data_type=Fixed-point  const_n_bits=29  const_bin_pt=28  float_type=Single  exp_bits=8  fraction_bits=24  en=off  latency=0  precision=Full  arith_type="Signed  (2's comp)"  n_bits=16  bin_pt=14  quantization=Truncate  overflow=Wrap  use_behavioral_HDL=off  mem_type=Distributed RAM  pipeline=off  XmcBlockStatus=1  maskContainerNames=tabcontainer1  block_type=cmult  block_config=sysgen:CMult_config
      settings: infoedit=[]
  Cast2 : hdlBasic/Convert  Commented=on  gui_display_data_type=Fixed-point  arith_type=Unsigned  n_bits=8  bin_pt=7  float_type=Double  exp_bits=8  fraction_bits=24  quantization="Round  (unbiased: +/- Inf)"  overflow=Saturate  en=off  latency=0  pipeline=on  XmcBlockStatus=1  maskContainerNames=group2  block_type=convert  block_config=sysgen:Convert_config
  Gate_In1 : hdlBasic/Gateway In  gui_display_data_type=Fixed-point  arith_type=Signed (2's comp)  n_bits=29  bin_pt=27  preci_type=Double  exp_width=8  frac_width=24  rows=1  columns=1  quantization=Truncate  overflow=Wrap  period=1  UseAsADC=off  ADCChannel='1'  interface=None  automatic_assignment=on  address_offset=hex2dec('00')  intf_name=''  intf_description=''  default_value=0  timing_constraint=None  locs_specified=off  LOCs={}  io_standard={}  inherit_from_input=off  hdl_port=on  XmcBlockStatus=1  maskContainerNames=group4  block_type=gatewayin  block_config=sysgen:gateway_in_config  block_width_w=590  block_height_w=620  block_width=640  block_height=850
  Gate_In2 : hdlBasic/Gateway In  gui_display_data_type=Fixed-point  arith_type=Signed (2's comp)  n_bits=29  bin_pt=27  preci_type=Double  exp_width=8  frac_width=24  rows=1  columns=1  quantization=Truncate  overflow=Wrap  period=1  UseAsADC=off  ADCChannel='1'  interface=None  automatic_assignment=on  address_offset=hex2dec('00')  intf_name=''  intf_description=''  default_value=0  timing_constraint=None  locs_specified=off  LOCs={}  io_standard={}  inherit_from_input=off  hdl_port=on  XmcBlockStatus=1  maskContainerNames=group4  block_type=gatewayin  block_config=sysgen:gateway_in_config  block_width_w=590  block_height_w=620  block_width=640  block_height=850
  Gate_out1 : hdlBasic/Gateway Out  inherit_from_input=off  hdl_port=on  rows=1  columns=1  UseAsDAC=off  DACChannel='1'  interface=None  automatic_assignment=on  address_offset=hex2dec('00')  intf_name=''  intf_description=''  timing_constraint=None  locs_specified=off  LOCs={}  io_standard={}  XmcBlockStatus=1  maskContainerNames=group4  block_type=gatewayout  block_config=sysgen:gateway_out_config  block_width_w=590  block_height_w=620  block_width=620  block_height=750
  Mux : hdlBasic/Mux  inputs=2  en=off  latency=0  precision=Full  arith_type=Unsigned  n_bits=16  bin_pt=14  quantization=Truncate  overflow=Wrap  XmcBlockStatus=1  maskContainerNames=tabcontainer1  block_type=mux  block_config=sysgen:Mux_config
  Scale1 : hdlBasic/Scale  scale_factor=-28  XmcBlockStatus=1  maskContainerNames=group1  block_type=scale  block_config=sysgen:Scale_config
  Scale2 : hdlBasic/Scale  scale_factor=-27  XmcBlockStatus=1  maskContainerNames=group1  block_type=scale  block_config=sysgen:Scale_config
  Scale3 : hdlBasic/Scale  scale_factor=-28  XmcBlockStatus=1  maskContainerNames=group1  block_type=scale  block_config=sysgen:Scale_config
  Slice1 : hdlBasic/Slice  nbits=8  boolean_output=off  mode=Two Bit Locations  bit1=-1  base1=MSB of Input  bit0=28  base0=LSB of Input  XmcBlockStatus=1  maskContainerNames=group1  block_type=slice  block_config=sysgen:Slice_config
  Slice2 : hdlBasic/Slice  nbits=28  boolean_output=off  mode=Upper Bit Location + Width  bit1=-3  base1=MSB of Input  bit0=7  base0=LSB of Input  XmcBlockStatus=1  maskContainerNames=group1  block_type=slice  block_config=sysgen:Slice_config
  Slice3 : hdlBasic/Slice  nbits=7  boolean_output=off  mode=Two Bit Locations  bit1=-5  base1=MSB of Input  bit0=27  base0=LSB of Input  XmcBlockStatus=1  maskContainerNames=group1  block_type=slice  block_config=sysgen:Slice_config
  abs{1..4} (4 alike) : hdlBasic/Absolute  precision=Full  arith_type=Unsigned  n_bits=16  bin_pt=14  quantization=Truncate  overflow=Wrap  en=off  latency=0  XmcBlockStatus=1  maskContainerNames=tabcontainer1  block_type=abs  block_config=sysgen:Abs_config
  addsub1 : hdlBasic/AddSub  mode=Subtraction  use_carryin=off  use_carryout=off  en=off  latency=0  precision=Full  arith_type="Signed  (2's comp)"  n_bits=35  bin_pt=32  quantization="Round  (unbiased: +/- Inf)"  overflow=Saturate  use_behavioral_HDL=off  hw_selection=Fabric  pipelined=on  XmcBlockStatus=1  maskContainerNames=tabcontainer1  block_type=addsub  block_config=sysgen:Addsub_config
  addsub2 : hdlBasic/AddSub  mode=Addition  use_carryin=off  use_carryout=off  en=off  latency=0  precision=Full  arith_type=Unsigned  n_bits=16  bin_pt=14  quantization="Round  (unbiased: +/- Inf)"  overflow=Saturate  use_behavioral_HDL=off  hw_selection=Fabric  pipelined=on  XmcBlockStatus=1  maskContainerNames=tabcontainer1  block_type=addsub  block_config=sysgen:Addsub_config
  addsub3 : hdlBasic/AddSub  mode=Addition  use_carryin=off  use_carryout=off  en=off  latency=0  precision=Full  arith_type=Unsigned  n_bits=16  bin_pt=14  quantization="Round  (unbiased: +/- Inf)"  overflow=Saturate  use_behavioral_HDL=off  hw_selection=Fabric  pipelined=on  XmcBlockStatus=1  maskContainerNames=tabcontainer1  block_type=addsub  block_config=sysgen:Addsub_config
  addsub4 : hdlBasic/AddSub  mode=Addition  use_carryin=off  use_carryout=off  en=off  latency=0  precision=Full  arith_type=Unsigned  n_bits=17  bin_pt=16  quantization="Round  (unbiased: +/- Inf)"  overflow=Saturate  use_behavioral_HDL=off  hw_selection=Fabric  pipelined=on  XmcBlockStatus=1  maskContainerNames=tabcontainer1  block_type=addsub  block_config=sysgen:Addsub_config
  bool1 : hdlBasic/Relational  mode=a<b  op_type=Bool  en=off  latency=0  XmcBlockStatus=1  maskContainerNames=tabcontainer1  block_type=relational  block_config=sysgen:Relational_config
  mult3 : hdlBasic/Mult  Commented=on  precision=Full  arith_type="Signed  (2's comp)"  n_bits=16  bin_pt=14  quantization="Round  (unbiased: +/- Inf)"  overflow=Saturate  en=off  latency=0  use_behavioral_HDL=off  opt=Area  use_embedded=off  optimum_pipeline=off  pipeline=on  use_rpm=on  placement_style=Triangular  XmcBlockStatus=1  maskContainerNames=group1  block_type=mult  block_config=sysgen:Mult_config
  Out1 : Outport
  wires:
  addsub1/1 -> abs1/1
  abs1/1 -> addsub3/1
  CMult1/1 -> addsub2/1, addsub1/1
  CMult2/1 -> addsub2/2, addsub1/2
  CMult3/1 -> Slice1/1
  Mux/1 -> CMult3/1
  imx/1 -> Gate_In2/1
  Gate_out1/1 -> Out1/1
  rex/1 -> Gate_In1/1
  Slice1/1 -> Scale1/1
  bool1/1 -> Mux/1
  addsub3/1 -> Slice3/1
  addsub4/1 -> Slice2/1
  addsub2/1 -> abs2/1
  Gate_In2/1 -> abs4/1, CMult2/1
  Gate_In1/1 -> CMult1/1, abs3/1
  abs2/1 -> addsub3/2
  abs3/1 -> addsub4/1
  abs4/1 -> addsub4/2
  Scale1/1 -> Gate_out1/1
  Slice2/1 -> Scale2/1
  Scale3/1 -> bool1/1, Mux/2
  Scale2/1 -> Mux/3, bool1/2
  Slice3/1 -> Scale3/1
